simulink library "ddm"  (R2021b)
settings: Solver=VariableStepAuto  StartTime=0.0  StopTime=10.0  RelTol=1e-3
undefined symbols (not defined in the file or in its folder): ENUM_ADASACCSTA_ERROR, ENUM_ADASACCSTA_OFF, ENUM_ADASACCSTA_STANDBY, ENUM_ADASISASTA_OFF, ENUM_ALLOWMOV_ALLOWREADY, ENUM_APS, ENUM_BRKSTA_ERROR, ENUM_BRKSTA_OFF, ENUM_BRKSTA_ON, ENUM_BRKSW_INVALID, ENUM_BRKSW_OFF, ENUM_BRKSW_ON, ENUM_CHGPREACTERRSTA_OBCPRE, ENUM_DCDCFAULTSTA_ANYFAULTLV1, ENUM_DCDCFAULTSTA_ANYFAULTLV2, ENUM_DRIVETRAIN_AWD, ENUM_DRIVETRAIN_FWD, ENUM_DRIVETRAIN_RWD, ENUM_DRSEATSTA_INVALID, ENUM_EDUDRTSTA_NORMAL, ENUM_EPBSTA_APPLIED, ENUM_EPBSTA_RELEASED, ENUM_HVBATTREADYPRE_READY, ENUM_MCUWARN_LV0, ENUM_MCUWARN_LV1, ENUM_MCUWARN_LV2, ENUM_MCUWARN_LV3, ENUM_MCUWARN_NOERROR, ENUM_OBCFAULTSTA_ANYFAULT, ENUM_PAS_R2F2, ENUM_PDFAULT_BATTPDFAIL, ENUM_PDFAULT_DCDCDISABLE, ENUM_PDFAULT_MCUDISABLE, ENUM_PDFAULT_MCUDISCHRG, ENUM_POWERSTA_OFF, ENUM_POWERSTA_ON, ENUM_POWERSTA_READY, ENUM_POWERSTA_STANDBY, ENUM_PRESSINDI_LOW, ENUM_PUFAULT_BATTUPFAIL, ENUM_PUFAULT_DCDCENABLEFAIL, ENUM_PUFAULT_PRECHRGCHKFAIL, ENUM_PUFAULT_SAFETYCHKFAIL, ENUM_PUSTATE_COMPLETED, ENUM_PWRSTASW_OFF, ENUM_PWRSTASW_OFFA, ENUM_PWRSTASW_OFFCHVCHRG, ENUM_PWRSTASW_OFFCLVCHRG, ENUM_PWRSTASW_ON, ENUM_PWRSTASW_ONHVCHRG, ENUM_PWRSTASW_READY, ENUM_PWRSTASW_STANDBY, ENUM_RANGESTA_12IN, ENUM_SHIFTCOMMAND_D, ENUM_SHIFTCOMMAND_N, ENUM_SHIFTCOMMAND_P, ENUM_SHIFTCOMMAND_R, ENUM_VEHMALFUNLV_2ND, ENUM_VEHMALFUNLV_3RD, ENUM_VEHMALFUNLV_4TH ... (+835)
libraries: hcu_lib x750, $bdroot x12, simulink x5
(part 10 of 28)

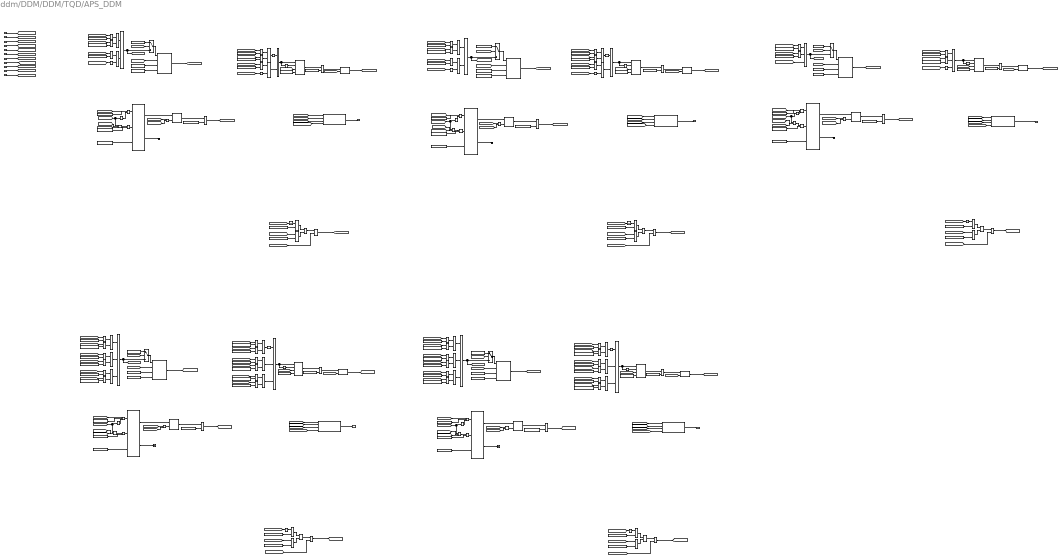
== system ddm/DDM/DDM/TQD/APS_DDM ==
  note: APS2 5V Out of Range (5vAPS2PwrErr)
  note: APS2 Signal Out of Range (APS2SigOoR)
  note: APS Correlation Error (APSCorrErr)
  note: APS1 5V Out of Range (5vAPS1PwrErr)
  note: APS1 Signal Out of Range (APS1SigOoR)
  VPMM_SysPwrSta_enum : Inport
  VINP_AccelPedal1Vol_V : Inport  Port=2
  VINP_AccelPedal2Vol_V : Inport  Port=3
  VDHP_EAPS12RangeSta_enum : Inport  Port=4
  VDHP_EAPCRBAD_flg : Inport  Port=5
  VINP_Pedal1Ref5V_V : Inport  Port=6
  VINP_Pedal2Ref5V_V : Inport  Port=7
  VINP_HVBattSOC_pct : Inport  Port=8
  task_time_s : Inport  Port=9
  DTC_clear_request : Inport  Port=10
  VDDM_AuxBattVolV_V : Inport  Port=11
  Constant{1,10,26,59,94} (5 alike) : Constant  Value=ENUM_POWERSTA_OFF
  Constant{62,65,84,92,100,103} (6 alike) : Constant  Value=ENUM_PWRSTASW_OFF
  Constant101 : Constant  Value=KDDM_APS2SigOoRHiLim_V
  Constant102 : Constant  Value=KDDM_APS2SigOoRLoLim_V
  Constant104 : Constant  Value=KDDM_APS2SigOoRHiLim_V
  Constant105 : Constant  Value=KDDM_APS2SigOoRLoLim_V
  Constant{2,11,76,95,106} (5 alike) : Constant  Value=ENUM_POWERSTA_STANDBY
  Constant107 : Constant  Value=KDDM_APS2SigOoRPassTO_s
  Constant108 : Constant  Value=KDDM_APS2SigOoRPassTO_s
  Constant109 : Constant  Value=KDDM_5vAPS2PwrErrPassTO_s
  Constant110 : Constant  Value=KDDM_APS2SigOoRCFSSW_flg
  Constant{21,85,90,99,111} (5 alike) : Constant  Value=FALSE
  Constant112 : Constant  Value=KDDM_5vAPS2PwrErrDetTO_s
  Constant113 : Constant  Value=KDDM_5vAPS2PwrErrCFSSW_flg
  Constant116 : Constant  Value=KDDM_5vAPS2PwrErrDetSW_flg
  Constant117 : Constant  Value=KDDM_5vAPS2PwrErrPassSW_flg
  Constant118 : Constant  Value=KDDM_5vAPS2PwrErrDTC_cnt
  Constant119 : Constant  Value=KDDM_5vAPS2PwrErrDTC_cnt
  Constant12 : Constant  Value=KDDM_APS1SigOoRDetSW_flg
  Constant13 : Constant  Value=KDDM_APS1SigOoRPassSW_flg
  Constant132 : Constant  Value=KDDM_APS1SigOoRDTC_cnt
  Constant14 : Constant  Value=KDDM_APS1SigOoRDTC_cnt
  Constant15 : Constant  Value=KDDM_APS2SigOoRDTC_cnt
  Constant{16,24,27,35} (4 alike) : Constant  Value=KDDM_LVBattHiLim_V
  Constant{17,28,31,36} (4 alike) : Constant  Value=KDDM_LVBattLoLim_V
  Constant{18,29,32,37} (4 alike) : Constant  Value=ENUM_PWRSTASW_READY
  Constant19 : Constant  Value=KDDM_5vAPS1PwrErrPassTO_s
  Constant20 : Constant  Value=KDDM_5vAPS1PwrErrPassTO_s
  Constant22 : Constant  Value=KDDM_5vAPS1PwrErrDetTO_s
  Constant23 : Constant  Value=KDDM_5vAPS1PwrErrCFSSW_flg
  Constant{7,25,38,41} (4 alike) : Constant  Value=ENUM_PWRSTASW_ON
  Constant3 : Constant  Value=KDDM_5vAPS1PwrErrDetSW_flg
  Constant30 : Constant  Value=KDDM_5vAPS2PwrErrPassTO_s
  Constant{8,33,39,42} (4 alike) : Constant  Value=KDDM_5vAPS1PwrErrHiLim_V
  Constant{9,34,40,43} (4 alike) : Constant  Value=KDDM_5vAPS1PwrErrLoLim_V
  Constant4 : Constant  Value=KDDM_5vAPS1PwrErrPassSW_flg
  Constant5 : Constant  Value=KDDM_5vAPS1PwrErrDTC_cnt
  Constant55 : Constant  Value=KDDM_APSCorrErrPassTO_s
  Constant56 : Constant  Value=ENUM_RANGESTA_12IN
  Constant57 : Constant  Value=KDDM_APSCorrErrDetTO_s
  Constant58 : Constant  Value=KDDM_APSCorrErrDTC_cnt
  Constant6 : Constant  Value=KDDM_5vAPS1PwrErrDTC_cnt
  Constant63 : Constant  Value=KDDM_APS1SigOoRHiLim_V
  Constant64 : Constant  Value=KDDM_APS1SigOoRLoLim_V
  Constant66 : Constant  Value=KDDM_APS1SigOoRHiLim_V
  Constant67 : Constant  Value=KDDM_APS1SigOoRLoLim_V
  Constant68 : Constant  Value=KDDM_APS2SigOoRDetTO_s
  Constant69 : Constant  Value=KDDM_APS1SigOoRPassTO_s
  Constant70 : Constant  Value=KDDM_APS1SigOoRPassTO_s
  Constant71 : Constant  Value=KDDM_APSCorrErrCFSSW_flg
  Constant83 : Constant  Value=ENUM_RANGESTA_12IN
  Constant86 : Constant  Value=KDDM_APS1SigOoRDetTO_s
  Constant87 : Constant  Value=KDDM_APSCorrErrDetSW_flg
  Constant88 : Constant  Value=KDDM_APSCorrErrPassSW_flg
  Constant89 : Constant  Value=KDDM_APSCorrErrDTC_cnt
  Constant91 : Constant  Value=KDDM_APSCorrErrPassTO_s
  Constant93 : Constant  Value=KDDM_APS1SigOoRCFSSW_flg
  Constant96 : Constant  Value=KDDM_APS2SigOoRDetSW_flg
  Constant97 : Constant  Value=KDDM_APS2SigOoRPassSW_flg
  Constant98 : Constant  Value=KDDM_APS2SigOoRDTC_cnt
  DTC_Couter{1..5} (5 alike) : hcu_lib/Basic_Blocks/DTC_Couter
  DTC_Info{,1..4} (5 alike) : hcu_lib/Basic_Blocks/DTC_Info
  Equal{1,3..4,6..7,10..12,14..17,36..37,56..57,66..67,74..75} (20 alike) : RelationalOperator  Operator===  OutDataTypeStr=boolean  RndMeth=Simplest
  Equal{5,13,19,23,26..27,29,31,33,35,60,63} (12 alike) : RelationalOperator  Operator=<  OutDataTypeStr=boolean  RndMeth=Simplest
  Equal{2,8,18,20,22,25,30,32,34,38,59,62} (12 alike) : RelationalOperator  Operator=>  OutDataTypeStr=boolean  RndMeth=Simplest
  Equal{21,24,51,53,58,61} (6 alike) : RelationalOperator  Operator=~=  OutDataTypeStr=boolean  RndMeth=Simplest
  Equal{9,28,55,65,70} (5 alike) : RelationalOperator  OutDataTypeStr=boolean  RndMeth=Simplest
  Logical Operator{1..2,8,10,12..14,19,26..27,33,37,41,48,50,52,54,56,80,97,103,110} (22 alike) : Logic  Operator=OR  AllPortsSameDT=off  OutDataTypeStr=boolean
  Logical Operator{4,6..7,9,16..18,20,24,30..32,34,38..39,47,59,72,82,85,100..102,107..109,116} (27 alike) : Logic  AllPortsSameDT=off  OutDataTypeStr=boolean
  Logical Operator{22,28..29,36,40,42,45,49,51,53,55,62,71,73,83,98,105,111..112} (19 alike) : Logic  Operator=NOT  AllPortsSameDT=off  OutDataTypeStr=boolean
  Logical Operator{11,15,35,43,60} (5 alike) : Logic  Operator=OR  Inputs=3  AllPortsSameDT=off  OutDataTypeStr=boolean
  Logical Operator{3,5,21,23,25,44,46,70,84,86,115} (11 alike) : Logic  Inputs=3  AllPortsSameDT=off  OutDataTypeStr=boolean
  SR_Latch{,1..4,6,12,15,18,20} (10 alike) : hcu_lib/Basic_Blocks/SR_Latch
  Switch{1..4,6} (5 alike) : Switch  Criteria=u2 ~= 0
  Terminator{,1..4} (5 alike) : Terminator
  Test Detection Criteria{1..5} (5 alike) : hcu_lib/Basic_Blocks/Test Detection Criteria
  Timer{1,4..5,13,15} (5 alike) : hcu_lib/Basic_Blocks/Timer
  Unit Delay{,1..2,5,7} (5 alike) : UnitDelay  SampleTime=-1  HasFrameUpgradeWarning=on
  VDDM_APS1SigOoRDTC_raw32 : Outport
  VDDM_APS2SigOoRDTC_raw32 : Outport  Port=2
  VDDM_APSCorrErrDTC_raw32 : Outport  Port=3
  VDDM_5vAPS1PwrErrDTC_raw32 : Outport  Port=4
  VDDM_5vAPS2PwrErrDTC_raw32 : Outport  Port=5
  wires:
  Logical Operator56/1 -> SR_Latch3/2
  [DTC_clear_request] -> Logical Operator56/2
  [DTC_clear_request] -> Logical Operator15/1, Logical Operator55/1
  Logical Operator55/1 -> Logical Operator21/3
  [DTC_clear_request] -> Logical Operator54/2
  Logical Operator54/1 -> SR_Latch1/2
  [DTC_clear_request] -> Logical Operator53/1, Logical Operator11/1
  Logical Operator53/1 -> Logical Operator23/3
  [DTC_clear_request] -> Logical Operator52/2
  Logical Operator52/1 -> SR_Latch12/2
  [DTC_clear_request] -> Logical Operator51/1, Logical Operator60/1
  Logical Operator51/1 -> Logical Operator84/3
  [DTC_clear_request] -> Logical Operator50/2
  Logical Operator50/1 -> SR_Latch6/2
  [DTC_clear_request] -> Logical Operator49/1, Logical Operator43/1
  Logical Operator49/1 -> Logical Operator115/3
  [DTC_clear_request] -> Logical Operator37/2
  Logical Operator37/1 -> SR_Latch/2
  Logical Operator29/1 -> Logical Operator5/3
  [DTC_clear_request] -> Logical Operator29/1, Logical Operator35/1
  Logical Operator45/1 -> Logical Operator46/1
  Logical Operator48/1 -> Logical Operator46/2
  [VPMM_SysPwrSta_enum] -> Equal37/1
  Equal36/1 -> Logical Operator48/1
  Constant43/1 -> Equal35/2
  Constant41/1 -> Equal36/2
  Equal35/1 -> Logical Operator14/2
  Equal34/1 -> Logical Operator14/1
  Equal37/1 -> Logical Operator48/2
  Logical Operator47/1 -> Logical Operator46/3
  Constant29/1 -> Equal37/2
  [VPMM_SysPwrSta_enum] -> Equal36/1
  [VINP_Pedal2Ref5V_V] -> Equal34/1
  Logical Operator14/1 -> Logical Operator45/1
  Equal27/1 -> Logical Operator47/2
  Constant28/1 -> Equal38/2
  Equal38/1 -> Logical Operator47/1
  Constant42/1 -> Equal34/2
  [VINP_Pedal2Ref5V_V] -> Equal35/1
  Constant27/1 -> Equal27/2
  [VDDM_AuxBattVolV_V] -> Equal38/1
  [VDDM_AuxBattVolV_V] -> Equal27/1
  [VDDM_AuxBattVolV_V] -> Equal31/1
  [VDDM_AuxBattVolV_V] -> Equal30/1
  Equal30/1 -> Logical Operator20/1
  Constant35/1 -> Equal31/2
  [VINP_Pedal2Ref5V_V] -> Equal33/1
  Constant36/1 -> Equal30/2
  Constant39/1 -> Equal32/2
  Logical Operator20/1 -> Logical Operator44/3
  Equal17/1 -> Logical Operator26/2
  Equal31/1 -> Logical Operator20/2
  [VINP_Pedal2Ref5V_V] -> Equal32/1
  Constant37/1 -> Equal17/2
  [VPMM_SysPwrSta_enum] -> Equal14/1
  Logical Operator27/1 -> Logical Operator44/1
  Equal32/1 -> Logical Operator27/1
  Equal33/1 -> Logical Operator27/2
  Constant38/1 -> Equal14/2
  Constant40/1 -> Equal33/2
  [VPMM_SysPwrSta_enum] -> Equal17/1
  Equal14/1 -> Logical Operator26/1
  Logical Operator26/1 -> Logical Operator44/2
  Logical Operator22/1 -> Logical Operator25/1
  Logical Operator10/1 -> Logical Operator22/1
  [VDDM_AuxBattVolV_V] -> Equal13/1
  [VDDM_AuxBattVolV_V] -> Equal8/1
  Equal8/1 -> Logical Operator7/1
  Constant16/1 -> Equal13/2
  [VINP_Pedal1Ref5V_V] -> Equal29/1
  Constant17/1 -> Equal8/2
  Constant33/1 -> Equal20/2
  Logical Operator7/1 -> Logical Operator25/3
  Equal7/1 -> Logical Operator8/2
  Equal13/1 -> Logical Operator7/2
  [VINP_Pedal1Ref5V_V] -> Equal20/1
  Constant18/1 -> Equal7/2
  [VPMM_SysPwrSta_enum] -> Equal6/1
  Equal20/1 -> Logical Operator10/1
  Equal29/1 -> Logical Operator10/2
  Constant25/1 -> Equal6/2
  Constant34/1 -> Equal29/2
  [VPMM_SysPwrSta_enum] -> Equal7/1
  Equal6/1 -> Logical Operator8/1
  Logical Operator8/1 -> Logical Operator25/2
  Constant32/1 -> Equal12/2
  [VPMM_SysPwrSta_enum] -> Equal12/1
  Equal12/1 -> Logical Operator19/2
  Logical Operator19/1 -> Logical Operator3/2
  Equal1/1 -> Logical Operator19/1
  Equal18/1 -> Logical Operator18/1
  Equal19/1 -> Logical Operator18/2
  Logical Operator18/1 -> Logical Operator3/3
  Constant31/1 -> Equal18/2
  Constant24/1 -> Equal19/2
  [VDDM_AuxBattVolV_V] -> Equal18/1
  [VDDM_AuxBattVolV_V] -> Equal19/1
  VDDM_AuxBattVolV_V/1 -> [VDDM_AuxBattVolV_V]
  Logical Operator44/1 -> Switch4/3, [VDDM_5vAPS2PwrErrRst_flg]
  DTC_Couter5/1 -> SR_Latch3/1
  Logical Operator16/1 -> Logical Operator13/1
  Logical Operator15/1 -> Logical Operator59/1
  Equal70/1 -> SR_Latch4/1
  Timer5/1 -> Equal70/1
  Test Detection Criteria5/1 -> [VDDM_5vAPS2PwrErrDet_flg]  "VDDM_5vAPS2PwrErrDet_flg"
  Logical Operator62/1 -> Timer5/2
  [VDDM_5vAPS2PwrErrDet_flg] -> Logical Operator21/1
  DTC_Info4/1 -> VDDM_5vAPS2PwrErrDTC_raw32/1  "VDDM_5vAPS2PwrErrDTC_raw32"
  SR_Latch4/1 -> [VDDM_5vAPS2PwrErrPass_flg]  "VDDM_5vAPS2PwrErrPass_flg"
  [VDDM_5vAPS2PwrErrCFSRls_flg] -> Logical Operator15/2
  [VDDM_5vAPS2PwrErrCFS_flg] -> DTC_Info4/3
  Constant116/1 -> Logical Operator21/2
  Logical Operator59/1 -> DTC_Couter5/2
  Constant109/1 -> Timer5/4
  Constant111/1 -> Switch4/1
  [DTC_clear_request] -> DTC_Info4/4
  Constant113/1 -> Logical Operator72/2
  [VPMM_SysPwrSta_enum] -> Equal16/1
  [task_time_s] -> Timer5/3
  Constant26/1 -> Equal15/2
  Constant118/1 -> Test Detection Criteria5/3
  [task_time_s] -> Test Detection Criteria5/2
  Constant119/1 -> DTC_Couter5/3
  Constant106/1 -> Equal16/2
  SR_Latch3/1 -> Logical Operator72/1
  Equal15/1 -> Logical Operator16/1
  [VDDM_5vAPS2PwrErrPass_flg] -> DTC_Info4/2
  Constant30/1 -> Equal70/2
  Unit Delay2/1 -> Equal15/1
  [VPMM_SysPwrSta_enum] -> Unit Delay2/1
  [DTC_clear_request] -> Logical Operator13/2
  [DTC_clear_request] -> Switch4/2
  Logical Operator13/1 -> [VDDM_5vAPS2PwrErrCFSRls_flg]  "VDDM_5vAPS2PwrErrCFSRls_flg"
  Constant117/1 -> Logical Operator59/2
  Constant112/1 -> Test Detection Criteria5/4
  Equal16/1 -> Logical Operator16/2
  [VDDM_5vAPS2PwrErrRst_flg] -> SR_Latch4/2
  [VDDM_5vAPS2PwrErrCFSRls_flg] -> Logical Operator56/1
  Logical Operator21/1 -> DTC_Couter5/1
  Logical Operator72/1 -> [VDDM_5vAPS2PwrErrCFS_flg]  "VDDM_5vAPS2PwrErrCFS_flg"
  DTC_Couter5/2 -> Terminator4/1  "VDDM_5vAPS2PwrErrDTC_cnt"
  Logical Operator46/1 -> Logical Operator62/1, Timer5/1
  [VDDM_5vAPS2PwrErrDet_flg] -> DTC_Info4/1
  Switch4/1 -> Test Detection Criteria5/1
  [VDDM_5vAPS2PwrErrPass_flg] -> Logical Operator15/3
  VINP_HVBattSOC_pct/1 -> [VINP_HVBattSOC_pct]
  [VINP_Pedal1Ref5V_V] -> Equal5/1
  [VINP_Pedal1Ref5V_V] -> Equal2/1
  Logical Operator3/1 -> Switch3/3, [VDDM_5vAPS1PwrErrRst_flg]
  Constant9/1 -> Equal5/2
  [VPMM_SysPwrSta_enum] -> Equal1/1
  Constant8/1 -> Equal2/2
  Logical Operator2/1 -> Logical Operator3/1
  Equal5/1 -> Logical Operator2/2
  Equal2/1 -> Logical Operator2/1
  Constant7/1 -> Equal1/2
  Logical Operator1/1 -> [VDDM_5vAPS1PwrErrCFSRls_flg]  "VDDM_5vAPS1PwrErrCFSRls_flg"
  Logical Operator17/1 -> Logical Operator1/1
  SR_Latch2/1 -> [VDDM_5vAPS1PwrErrPass_flg]  "VDDM_5vAPS1PwrErrPass_flg"
  Logical Operator9/1 -> [VDDM_5vAPS1PwrErrCFS_flg]  "VDDM_5vAPS1PwrErrCFS_flg"
  Constant21/1 -> Switch3/1
  Logical Operator25/1 -> Logical Operator40/1, Timer4/1
  [task_time_s] -> Timer4/3
  Switch3/1 -> Test Detection Criteria2/1
  DTC_Info3/1 -> VDDM_5vAPS1PwrErrDTC_raw32/1  "VDDM_5vAPS1PwrErrDTC_raw32"
  [VPMM_SysPwrSta_enum] -> Equal11/1
  [DTC_clear_request] -> DTC_Info3/4
  Constant6/1 -> DTC_Couter4/3
  [task_time_s] -> Test Detection Criteria2/2
  [VPMM_SysPwrSta_enum] -> Unit Delay1/1
  SR_Latch1/1 -> Logical Operator9/1
  Equal10/1 -> Logical Operator17/1
  Constant2/1 -> Equal11/2
  Constant1/1 -> Equal10/2
  Constant5/1 -> Test Detection Criteria2/3
  DTC_Couter4/2 -> Terminator3/1  "VDDM_5vAPS1PwrErrDTC_cnt"
  [VDDM_5vAPS1PwrErrPass_flg] -> DTC_Info3/2
  [DTC_clear_request] -> Logical Operator1/2
  Logical Operator23/1 -> DTC_Couter4/1
  Constant19/1 -> Equal9/2
  Unit Delay1/1 -> Equal10/1
  Constant4/1 -> Logical Operator24/2
  Constant3/1 -> Logical Operator23/2
  [DTC_clear_request] -> Switch3/2
  [VDDM_5vAPS1PwrErrPass_flg] -> Logical Operator11/3
  DTC_Couter4/1 -> SR_Latch1/1
  Test Detection Criteria2/1 -> [VDDM_5vAPS1PwrErrDet_flg]  "VDDM_5vAPS1PwrErrDet_flg"
  Logical Operator11/1 -> Logical Operator24/1
  Equal11/1 -> Logical Operator17/2
  Logical Operator24/1 -> DTC_Couter4/2
  [VDDM_5vAPS1PwrErrCFSRls_flg] -> Logical Operator11/2
  Equal9/1 -> SR_Latch2/1
  Logical Operator40/1 -> Timer4/2
  Constant20/1 -> Timer4/4
  Timer4/1 -> Equal9/1
  [VDDM_5vAPS1PwrErrDet_flg] -> Logical Operator23/1
  Constant23/1 -> Logical Operator9/2
  Constant22/1 -> Test Detection Criteria2/4
  [VDDM_5vAPS1PwrErrRst_flg] -> SR_Latch2/2
  [VDDM_5vAPS1PwrErrDet_flg] -> DTC_Info3/1
  [VDDM_5vAPS1PwrErrCFS_flg] -> DTC_Info3/3
  [VDDM_5vAPS1PwrErrCFSRls_flg] -> Logical Operator54/1
  VINP_Pedal2Ref5V_V/1 -> [VINP_Pedal2Ref5V_V]
  VINP_Pedal1Ref5V_V/1 -> [VINP_Pedal1Ref5V_V]
  [VDDM_APSCorrErrRst_flg] -> SR_Latch20/2
  [VDDM_APS2SigOoRRst_flg] -> SR_Latch15/2
  [VDDM_APS1SigOoRRst_flg] -> SR_Latch18/2
  Logical Operator60/1 -> Logical Operator85/1
  [VDDM_APSCorrErrPass_flg] -> Logical Operator60/3
  [VDDM_APSCorrErrCFSRls_flg] -> Logical Operator60/2
  Logical Operator43/1 -> Logical Operator116/1
  [VDDM_APS2SigOoRPass_flg] -> Logical Operator43/3
  [VDDM_APS2SigOoRCFSRls_flg] -> Logical Operator43/2
  Logical Operator35/1 -> Logical Operator6/1
  [VDDM_APS1SigOoRCFSRls_flg] -> Logical Operator35/2
  [VDDM_APS1SigOoRPass_flg] -> Logical Operator35/3
  Constant99/1 -> Switch2/1
  Logical Operator86/1 -> Switch2/3, [VDDM_APSCorrErrRst_flg]
  Switch2/1 -> Test Detection Criteria1/1
  [DTC_clear_request] -> Switch2/2
  Constant90/1 -> Switch1/1
  Logical Operator101/1 -> Switch1/3, [VDDM_APS2SigOoRRst_flg]
  Switch1/1 -> Test Detection Criteria4/1
  [DTC_clear_request] -> Switch1/2
  Constant85/1 -> Switch6/1
  Logical Operator31/1 -> Switch6/3, [VDDM_APS1SigOoRRst_flg]
  Switch6/1 -> Test Detection Criteria3/1
  [DTC_clear_request] -> Switch6/2
  [DTC_clear_request] -> DTC_Info2/4
  [DTC_clear_request] -> DTC_Info1/4
  [DTC_clear_request] -> DTC_Info/4
  Logical Operator34/1 -> [VDDM_APSCorrErrCFS_flg]  "VDDM_APSCorrErrCFS_flg"
  SR_Latch12/1 -> Logical Operator34/1
  Constant71/1 -> Logical Operator34/2
  VDHP_EAPCRBAD_flg/1 -> [VDHP_EAPCRBAD_flg]
  VDHP_EAPS12RangeSta_enum/1 -> [VDHP_EAPS12RangeSta_enum]
  DTC_Info2/1 -> VDDM_APSCorrErrDTC_raw32/1  "VDDM_APSCorrErrDTC_raw32"
  [VDDM_APSCorrErrCFS_flg] -> DTC_Info2/3
  DTC_Couter3/2 -> Terminator2/1  "VDDM_APSCorrErrDTC_cnt"
  DTC_Couter3/1 -> SR_Latch12/1
  Constant89/1 -> DTC_Couter3/3
  Constant58/1 -> Test Detection Criteria1/3
  VINP_AccelPedal2Vol_V/1 -> [VINP_AccelPedal2Vol_V]
  VINP_AccelPedal1Vol_V/1 -> [VINP_AccelPedal1Vol_V]
  VPMM_SysPwrSta_enum/1 -> [VPMM_SysPwrSta_enum]
  DTC_Info1/1 -> VDDM_APS2SigOoRDTC_raw32/1  "VDDM_APS2SigOoRDTC_raw32"
  [VDDM_APS2SigOoRCFS_flg] -> DTC_Info1/3
  SR_Latch6/1 -> Logical Operator102/1
  [VDDM_APS2SigOoRCFSRls_flg] -> Logical Operator50/1
  DTC_Couter2/1 -> SR_Latch6/1
  DTC_Couter2/2 -> Terminator1/1  "VDDM_APS2SigOoRDTC_cnt"
  Constant98/1 -> DTC_Couter2/3
  Logical Operator116/1 -> DTC_Couter2/2
  Logical Operator115/1 -> DTC_Couter2/1
  Constant68/1 -> Test Detection Criteria4/4
  Constant15/1 -> Test Detection Criteria4/3
  [task_time_s] -> Test Detection Criteria4/2
  DTC_Couter1/2 -> Terminator/1  "VDDM_APS1SigOoRDTC_cnt"
  Equal28/1 -> SR_Latch18/1
  Logical Operator39/1 -> Logical Operator73/1, Timer1/1
  [VDDM_APS1SigOoRCFSRls_flg] -> Logical Operator37/1
  DTC_Couter1/1 -> SR_Latch/1
  Constant14/1 -> DTC_Couter1/3
  Logical Operator6/1 -> DTC_Couter1/2
  Logical Operator5/1 -> DTC_Couter1/1
  DTC_Info/1 -> VDDM_APS1SigOoRDTC_raw32/1  "VDDM_APS1SigOoRDTC_raw32"
  [VDDM_APS1SigOoRPass_flg] -> DTC_Info/2
  [VDDM_APS1SigOoRCFS_flg] -> DTC_Info/3
  Test Detection Criteria3/1 -> [VDDM_APS1SigOoRDet_flg]  "VDDM_APS1SigOoRDet_flg"
  Constant132/1 -> Test Detection Criteria3/3
  Constant86/1 -> Test Detection Criteria3/4
  [task_time_s] -> Test Detection Criteria3/2
  Logical Operator71/1 -> Logical Operator70/3
  [VDHP_EAPCRBAD_flg] -> Logical Operator71/1
  Constant84/1 -> Equal53/2
  [VPMM_SysPwrSta_enum] -> Equal53/1
  Constant56/1 -> Equal75/2
  Logical Operator70/1 -> Timer13/1, Logical Operator83/1
  [VDHP_EAPS12RangeSta_enum] -> Equal75/1
  Equal53/1 -> Logical Operator70/1
  Equal75/1 -> Logical Operator70/2
  Constant83/1 -> Equal74/2
  Equal74/1 -> Logical Operator86/2
  [VDHP_EAPS12RangeSta_enum] -> Equal74/1
  Equal55/1 -> SR_Latch20/1
  SR_Latch20/1 -> [VDDM_APSCorrErrPass_flg]  "VDDM_APSCorrErrPass_flg"
  [VDDM_5vAPS2PwrErrCFS_flg] -> Logical Operator98/1
  Logical Operator97/1 -> [VDDM_APS2SigOoRCFSRls_flg]  "VDDM_APS2SigOoRCFSRls_flg"
  [VINP_AccelPedal2Vol_V] -> Equal60/1
  [task_time_s] -> Timer15/3
  SR_Latch15/1 -> [VDDM_APS2SigOoRPass_flg]  "VDDM_APS2SigOoRPass_flg"
  Equal66/1 -> Logical Operator109/1
  Unit Delay7/1 -> Equal66/1
  Equal65/1 -> SR_Latch15/1
  [VDDM_APS2SigOoRDet_flg] -> Logical Operator115/1
  [VDDM_5vAPS2PwrErrCFS_flg] -> Logical Operator105/1
  Logical Operator105/1 -> Logical Operator107/2
  Constant105/1 -> Equal63/2
  [VINP_AccelPedal2Vol_V] -> Equal59/1
  [VINP_AccelPedal2Vol_V] -> Equal62/1
  Constant102/1 -> Equal60/2
  [VPMM_SysPwrSta_enum] -> Equal58/1
  [VPMM_SysPwrSta_enum] -> Equal61/1
  Equal60/1 -> Logical Operator103/2
  [VINP_AccelPedal2Vol_V] -> Equal63/1
  Equal63/1 -> Logical Operator110/2
  Timer15/1 -> Equal65/1
  Logical Operator112/1 -> Timer15/2
  Constant103/1 -> Equal61/2
  Constant108/1 -> Timer15/4
  Logical Operator111/1 -> Logical Operator108/1
  Equal62/1 -> Logical Operator110/1
  [VPMM_SysPwrSta_enum] -> Equal67/1
  Logical Operator102/1 -> [VDDM_APS2SigOoRCFS_flg]  "VDDM_APS2SigOoRCFS_flg"
  Constant110/1 -> Logical Operator102/2
  [VPMM_SysPwrSta_enum] -> Unit Delay7/1
  Constant107/1 -> Equal65/2
  Constant97/1 -> Logical Operator116/2
  Constant100/1 -> Equal58/2
  Constant96/1 -> Logical Operator115/2
  Equal59/1 -> Logical Operator103/1
  Logical Operator98/1 -> Logical Operator100/2
  Logical Operator110/1 -> Logical Operator111/1
  Constant104/1 -> Equal62/2
  Logical Operator109/1 -> Logical Operator97/1
  Constant101/1 -> Equal59/2
  Test Detection Criteria4/1 -> [VDDM_APS2SigOoRDet_flg]  "VDDM_APS2SigOoRDet_flg"
  Constant94/1 -> Equal66/2
  Equal58/1 -> Logical Operator100/1
  Logical Operator103/1 -> Logical Operator101/1
  Equal61/1 -> Logical Operator107/1
  Logical Operator107/1 -> Logical Operator108/2
  Equal67/1 -> Logical Operator109/2
  Logical Operator100/1 -> Logical Operator101/2
  Logical Operator108/1 -> Timer15/1, Logical Operator112/1
  Constant95/1 -> Equal67/2
  [DTC_clear_request] -> Logical Operator97/2
  SR_Latch18/1 -> [VDDM_APS1SigOoRPass_flg]  "VDDM_APS1SigOoRPass_flg"
  Constant93/1 -> Logical Operator32/2
  Logical Operator32/1 -> [VDDM_APS1SigOoRCFS_flg]  "VDDM_APS1SigOoRCFS_flg"
  SR_Latch/1 -> Logical Operator32/1
  [VDHP_EAPCRBAD_flg] -> Logical Operator86/3
  [VPMM_SysPwrSta_enum] -> Equal51/1
  Constant92/1 -> Equal51/2
  Equal51/1 -> Logical Operator86/1
  Constant76/1 -> Equal57/2
  Constant55/1 -> Timer13/4
  Constant87/1 -> Logical Operator84/2
  Logical Operator80/1 -> [VDDM_APSCorrErrCFSRls_flg]  "VDDM_APSCorrErrCFSRls_flg"
  [VDDM_APSCorrErrCFSRls_flg] -> Logical Operator52/1
  Logical Operator82/1 -> Logical Operator80/1
  [task_time_s] -> Test Detection Criteria1/2
  Constant91/1 -> Equal55/2
  Unit Delay5/1 -> Equal56/1
  Test Detection Criteria1/1 -> [VDDM_APSCorrErrDet_flg]  "VDDM_APSCorrErrDet_flg"
  Logical Operator83/1 -> Timer13/2
  Logical Operator84/1 -> DTC_Couter3/1
  Logical Operator85/1 -> DTC_Couter3/2
  Timer13/1 -> Equal55/1
  Constant88/1 -> Logical Operator85/2
  [VDDM_APSCorrErrDet_flg] -> Logical Operator84/1
  Constant59/1 -> Equal56/2
  [task_time_s] -> Timer13/3
  Constant57/1 -> Test Detection Criteria1/4
  [DTC_clear_request] -> Logical Operator80/2
  Equal57/1 -> Logical Operator82/2
  Equal56/1 -> Logical Operator82/1
  [VPMM_SysPwrSta_enum] -> Unit Delay5/1
  [VPMM_SysPwrSta_enum] -> Equal57/1
  [task_time_s] -> Timer1/3
  Constant70/1 -> Timer1/4
  Timer1/1 -> Equal28/1
  Constant69/1 -> Equal28/2
  Logical Operator73/1 -> Timer1/2
  Logical Operator42/1 -> Logical Operator39/1
  Logical Operator38/1 -> Logical Operator39/2
  Logical Operator36/1 -> Logical Operator38/2
  Equal24/1 -> Logical Operator38/1
  [VDDM_5vAPS1PwrErrCFS_flg] -> Logical Operator36/1
  Constant65/1 -> Equal24/2
  [VPMM_SysPwrSta_enum] -> Equal24/1
  Equal26/1 -> Logical Operator41/2
  Equal25/1 -> Logical Operator41/1
  Constant67/1 -> Equal26/2
  Constant66/1 -> Equal25/2
  [VINP_AccelPedal1Vol_V] -> Equal26/1
  [VINP_AccelPedal1Vol_V] -> Equal25/1
  Logical Operator41/1 -> Logical Operator42/1
  Logical Operator33/1 -> Logical Operator31/1
  [VINP_AccelPedal1Vol_V] -> Equal22/1
  [VINP_AccelPedal1Vol_V] -> Equal23/1
  Constant63/1 -> Equal22/2
  Constant64/1 -> Equal23/2
  Equal22/1 -> Logical Operator33/1
  Equal23/1 -> Logical Operator33/2
  [VPMM_SysPwrSta_enum] -> Equal21/1
  Constant62/1 -> Equal21/2
  [VDDM_5vAPS1PwrErrCFS_flg] -> Logical Operator28/1
  Equal21/1 -> Logical Operator30/1
  Logical Operator28/1 -> Logical Operator30/2
  Logical Operator30/1 -> Logical Operator31/2
  Logical Operator12/1 -> [VDDM_APS1SigOoRCFSRls_flg]  "VDDM_APS1SigOoRCFSRls_flg"
  Logical Operator4/1 -> Logical Operator12/1
  [DTC_clear_request] -> Logical Operator12/2
  Constant13/1 -> Logical Operator6/2
  Constant12/1 -> Logical Operator5/2
  [VDDM_APS1SigOoRDet_flg] -> Logical Operator5/1
  Equal4/1 -> Logical Operator4/2
  Equal3/1 -> Logical Operator4/1
  [VPMM_SysPwrSta_enum] -> Equal4/1
  Constant11/1 -> Equal4/2
  Constant10/1 -> Equal3/2
  Unit Delay/1 -> Equal3/1
  [VPMM_SysPwrSta_enum] -> Unit Delay/1
  task_time_s/1 -> [task_time_s]
  DTC_clear_request/1 -> [DTC_clear_request]
  [VDDM_APS1SigOoRDet_flg] -> DTC_Info/1
  [VDDM_APS2SigOoRDet_flg] -> DTC_Info1/1
  [VDDM_APS2SigOoRPass_flg] -> DTC_Info1/2
  [VDDM_APSCorrErrDet_flg] -> DTC_Info2/1
  [VDDM_APSCorrErrPass_flg] -> DTC_Info2/2

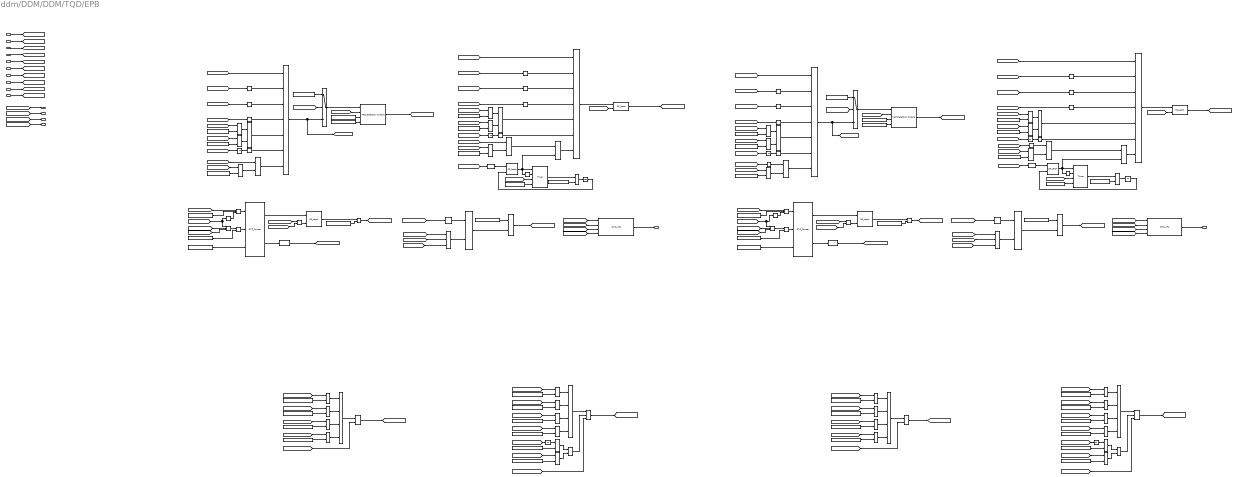
== system ddm/DDM/DDM/TQD/EPB ==
  note: EPB Release Response Timeout (EPBUnlockTO)
  note: EPB Apply Response Timeout (EPBLockTO)
  NO_CAN1_BUS_OFF : Inport
  CAN_LossOfEPB1 : Inport  Port=2
  RC_LossErrOfEPB1 : Inport  Port=3
  CS_LossErrOfEPB1 : Inport  Port=4
  VPMM_SysPwrSta_enum : Inport  Port=5
  VTQD_ActParkRequest_flg : Inport  Port=6
  VINP_EPBSta_enum : Inport  Port=7
  VINP_ShifterHandleCmd_enum : Inport  Port=8
  task_time_s : Inport  Port=9
  DTC_clear_request : Inport  Port=10
  AND{,1..5} (6 alike) : Logic  AllPortsSameDT=off  OutDataTypeStr=boolean
  Constant{,3,23,25} (4 alike) : Constant  Value=ENUM_PWRSTASW_ON
  Constant1 : Constant  Value=KDDM_EPBLockTOCFSSW_flg
  Constant{8,10,26,49} (4 alike) : Constant  Value=ENUM_PWRSTASW_READY
  Constant11 : Constant  Value=ENUM_EPBSTA_RELEASED
  Constant12 : Constant  Value=ENUM_POWERSTA_OFF
  Constant13 : Constant  Value=ENUM_POWERSTA_STANDBY
  Constant{14,29,41,45} (4 alike) : Constant  Value=ENUM_SHIFTCOMMAND_P
  Constant15 : Constant  Value=KDDM_EPBLockTODTC_cnt
  Constant16 : Constant  Value=KDDM_EPBLockTODFSSW_flg
  Constant{17,32,42,46} (4 alike) : Constant  Value=ENUM_SHIFTCOMMAND_N
  Constant{4,18,33,40} (4 alike) : Constant  Value=ENUM_SHIFTCOMMAND_D
  Constant{5,19,34,43} (4 alike) : Constant  Value=ENUM_SHIFTCOMMAND_R
  Constant2 : Constant  Value=FALSE
  Constant20 : Constant  Value=KDDM_EPBLockTODTC_cnt
  Constant21 : Constant  Value=KDDM_EPBUnlockTOPassTO_s
  Constant22 : Constant  Value=KDDM_EPBLockTODetTO_s
  Constant24 : Constant  Value=KDDM_EPBUnlockTOCFSSW_flg
  Constant27 : Constant  Value=ENUM_POWERSTA_OFF
  Constant28 : Constant  Value=ENUM_POWERSTA_STANDBY
  Constant30 : Constant  Value=KDDM_EPBUnlockTODTC_cnt
  Constant31 : Constant  Value=KDDM_EPBUnlockTODFSSW_flg
  Constant35 : Constant  Value=FALSE
  Constant36 : Constant  Value=KDDM_EPBUnlockTODTC_cnt
  Constant38 : Constant  Value=KDDM_EPBUnlockTODetTO_s
  Constant39 : Constant  Value=ENUM_EPBSTA_RELEASED
  Constant44 : Constant  Value=KDDM_EPBUnlockTODetSW_flg
  Constant47 : Constant  Value=KDDM_EPBUnlockTOPassSW_flg
  Constant50 : Constant  Value=ENUM_EPBSTA_APPLIED
  Constant51 : Constant  Value=ENUM_EPBSTA_APPLIED
  Constant52 : Constant  Value=KDDM_EPBLockTOPassTO_s
  Constant53 : Constant  Value=KDDM_EPBUnlockTOPassTO_s
  Constant6 : Constant  Value=KDDM_EPBLockTODetSW_flg
  Constant7 : Constant  Value=KDDM_EPBLockTOPassSW_flg
  Constant9 : Constant  Value=KDDM_EPBLockTOPassTO_s
  DTC_Couter1 : hcu_lib/Basic_Blocks/DTC_Couter
  DTC_Couter2 : hcu_lib/Basic_Blocks/DTC_Couter
  DTC_Info : hcu_lib/Basic_Blocks/DTC_Info
  DTC_Info1 : hcu_lib/Basic_Blocks/DTC_Info
  Data Type Conversion1 : DataTypeConversion  OutDataTypeStr=uint8
  Data Type Conversion2 : DataTypeConversion  OutDataTypeStr=uint8
  Detect Decrease : simulink/Logic and Bit Operations/Detect Decrease  vinit=0.0  OutDataTypeStr=boolean
  Detect Increase1 : simulink/Logic and Bit Operations/Detect Increase  vinit=0.0  OutDataTypeStr=boolean
  Equal{,1..2,4,6,8..26,28,30..34} (30 alike) : RelationalOperator  Operator===  OutDataTypeStr=boolean  RndMeth=Simplest
  Equal27 : RelationalOperator  Operator=~=  OutDataTypeStr=boolean  RndMeth=Simplest
  Equal3 : RelationalOperator  OutDataTypeStr=boolean  RndMeth=Simplest
  Equal5 : RelationalOperator  Operator=~=  OutDataTypeStr=boolean  RndMeth=Simplest
  Equal7 : RelationalOperator  OutDataTypeStr=boolean  RndMeth=Simplest
  Logical Operator{,4,6,8,25,29,49,51} (8 alike) : Logic  Operator=OR  AllPortsSameDT=off  OutDataTypeStr=boolean
  Logical Operator{1..2,9,16..18,24,55} (8 alike) : Logic  AllPortsSameDT=off  OutDataTypeStr=boolean
  Logical Operator{10..11,20,27,37,77} (6 alike) : Logic  Operator=OR  Inputs=3  AllPortsSameDT=off  OutDataTypeStr=boolean
  Logical Operator{12,14,23,28,30..36,38..39,41..48,50} (22 alike) : Logic  Operator=NOT  AllPortsSameDT=off  OutDataTypeStr=boolean
  Logical Operator13 : Logic  Inputs=3  AllPortsSameDT=off  OutDataTypeStr=boolean
  Logical Operator15 : Logic  Inputs=3  AllPortsSameDT=off  OutDataTypeStr=boolean
  Logical Operator{3,5,19,21} (4 alike) : Logic  Inputs=7  AllPortsSameDT=off  OutDataTypeStr=boolean
  Logical Operator{7,22,26,40} (4 alike) : Logic  Operator=OR  Inputs=4  AllPortsSameDT=off  OutDataTypeStr=boolean
  Relay1 : Relay  OnSwitchValue=ONE_INT  OffSwitchValue=ZERO_INT
  Relay2 : Relay  OnSwitchValue=ONE_INT  OffSwitchValue=ZERO_INT
  SR_Latch{1..8} (8 alike) : hcu_lib/Basic_Blocks/SR_Latch
  Switch1 : Switch  Criteria=u2 ~= 0
  Switch6 : Switch  Criteria=u2 ~= 0
  Test Detection Criteria1 : hcu_lib/Basic_Blocks/Test Detection Criteria
  Test Detection Criteria2 : hcu_lib/Basic_Blocks/Test Detection Criteria
  Timer2 : hcu_lib/Basic_Blocks/Timer
  Timer3 : hcu_lib/Basic_Blocks/Timer
  Unit Delay{,1..7} (8 alike) : UnitDelay  SampleTime=-1  HasFrameUpgradeWarning=on
  VDDM_EPBLockTODTC_raw32 : Outport
  VDDM_EPBUnlockTODTC_raw32 : Outport  Port=2
  VDDM_EPBLockTODFS_flg : Outport  Port=3
  VDDM_EPBLockTOCFS_flg : Outport  Port=4
  VDDM_EPBUnlockTODFS_flg : Outport  Port=5
  VDDM_EPBUnlockTOCFS_flg : Outport  Port=6
  wires:
  [DTC_clear_request] -> Logical Operator27/3
  [DTC_clear_request] -> Logical Operator51/2
  Logical Operator51/1 -> SR_Latch3/2
  [DTC_clear_request] -> Logical Operator50/1, Logical Operator10/1
  Logical Operator50/1 -> Logical Operator13/3
  [DTC_clear_request] -> Logical Operator77/3
  [DTC_clear_request] -> Logical Operator49/2
  Logical Operator49/1 -> SR_Latch1/2
  [DTC_clear_request] -> Logical Operator48/1, Logical Operator11/1
  Logical Operator48/1 -> Logical Operator15/3
  Unit Delay7/1 -> SR_Latch8/2
  Unit Delay6/1 -> SR_Latch7/2
  Logical Operator46/1 -> Logical Operator21/3
  [CS_LossErrOfEPB1] -> Logical Operator47/1
  Logical Operator47/1 -> Logical Operator21/4
  Logical Operator45/1 -> Logical Operator21/2
  [RC_LossErrOfEPB1] -> Logical Operator46/1
  [CAN_LossOfEPB1] -> Logical Operator45/1
  Logical Operator43/1 -> Logical Operator19/3
  [CS_LossErrOfEPB1] -> Logical Operator44/1
  Logical Operator44/1 -> Logical Operator19/4
  Logical Operator42/1 -> Logical Operator19/2
  [RC_LossErrOfEPB1] -> Logical Operator43/1
  [CAN_LossOfEPB1] -> Logical Operator42/1
  [CS_LossErrOfEPB1] -> Logical Operator41/1
  [RC_LossErrOfEPB1] -> Logical Operator39/1
  [CAN_LossOfEPB1] -> Logical Operator38/1
  Logical Operator41/1 -> Logical Operator5/4
  Logical Operator38/1 -> Logical Operator5/2
  Logical Operator39/1 -> Logical Operator5/3
  [RC_LossErrOfEPB1] -> Logical Operator35/1
  [CAN_LossOfEPB1] -> Logical Operator12/1
  Logical Operator35/1 -> Logical Operator3/3
  Logical Operator12/1 -> Logical Operator3/2
  Logical Operator36/1 -> Logical Operator3/4
  [CS_LossErrOfEPB1] -> Logical Operator36/1
  AND3/1 -> AND5/1
  AND5/1 -> Logical Operator21/7
  Logical Operator21/1 -> SR_Latch4/1
  Detect Decrease/1 -> SR_Latch8/1
  Constant53/1 -> Equal7/2
  SR_Latch8/1 -> Timer2/1, Logical Operator14/1, AND5/2
  [VTQD_ActParkRequest_flg] -> Detect Decrease/1
  Timer2/1 -> Equal7/1
  Equal7/1 -> Unit Delay7/1
  Constant21/1 -> Timer2/4
  [task_time_s] -> Timer2/3
  Logical Operator14/1 -> Timer2/2
  [VDDM_EPBLockTORst_flg] -> SR_Latch6/2
  SR_Latch6/1 -> [VDDM_EPBLockTOPass_flg]  "VDDM_EPBLockTOPass_flg"
  Logical Operator5/1 -> SR_Latch6/1
  AND1/1 -> Logical Operator5/7
  AND4/1 -> AND1/1
  Equal3/1 -> Unit Delay6/1
  Logical Operator34/1 -> Timer3/2
  SR_Latch7/1 -> Timer3/1, Logical Operator34/1, AND1/2
  Constant9/1 -> Equal3/2
  Timer3/1 -> Equal3/1
  Constant52/1 -> Timer3/4
  [task_time_s] -> Timer3/3
  [VTQD_ActParkRequest_flg] -> Detect Increase1/1
  Detect Increase1/1 -> SR_Latch7/1
  Constant51/1 -> Equal32/2
  Equal32/1 -> AND4/2
  [VTQD_ActParkRequest_flg] -> AND4/1
  [VINP_EPBSta_enum] -> Equal32/1
  DTC_clear_request/1 -> [DTC_clear_request]
  task_time_s/1 -> [task_time_s]
  VINP_ShifterHandleCmd_enum/1 -> [VINP_ShifterHandleCmd_enum]
  VINP_EPBSta_enum/1 -> [VINP_EPBSta_enum]
  VTQD_ActParkRequest_flg/1 -> [VTQD_ActParkRequest_flg]
  VPMM_SysPwrSta_enum/1 -> [VPMM_SysPwrSta_enum]
  CS_LossErrOfEPB1/1 -> [CS_LossErrOfEPB1]
  RC_LossErrOfEPB1/1 -> [RC_LossErrOfEPB1]
  CAN_LossOfEPB1/1 -> [CAN_LossOfEPB1]
  NO_CAN1_BUS_OFF/1 -> [NO_CAN1_BUS_OFF]
  [VTQD_ActParkRequest_flg] -> Logical Operator33/1
  Constant39/1 -> Equal23/2
  Equal23/1 -> AND3/2
  [VINP_EPBSta_enum] -> Equal23/1
  Logical Operator33/1 -> AND3/1
  Logical Operator32/1 -> AND2/1
  [VTQD_ActParkRequest_flg] -> Logical Operator32/1
  AND2/1 -> Logical Operator19/7
  [VINP_EPBSta_enum] -> Equal5/1
  Equal5/1 -> AND2/2
  Constant11/1 -> Equal5/2
  [VTQD_ActParkRequest_flg] -> AND/1
  Equal27/1 -> AND/2
  Constant50/1 -> Equal27/2
  [VINP_EPBSta_enum] -> Equal27/1
  Logical Operator19/1 -> Switch1/3, [VDDM_EPBUnlockTORst_flg]
  [VDDM_EPBLockTOCFS_flg] -> Unit Delay5/1
  Unit Delay5/1 -> Logical Operator23/1
  Logical Operator23/1 -> Logical Operator21/6
  [VPMM_SysPwrSta_enum] -> Equal26/1
  [VPMM_SysPwrSta_enum] -> Equal22/1
  Equal26/1 -> Logical Operator29/2
  [NO_CAN1_BUS_OFF] -> Logical Operator21/1
  Logical Operator29/1 -> Logical Operator21/5
  Equal22/1 -> Logical Operator29/1
  Constant26/1 -> Equal26/2
  Constant25/1 -> Equal22/2
  Constant23/1 -> Equal15/2
  Equal15/1 -> Logical Operator8/1
  Constant49/1 -> Equal16/2
  Equal16/1 -> Logical Operator8/2
  Logical Operator8/1 -> Logical Operator19/5
  [VPMM_SysPwrSta_enum] -> Equal15/1
  [NO_CAN1_BUS_OFF] -> Logical Operator19/1
  [VPMM_SysPwrSta_enum] -> Equal16/1
  [VDDM_EPBLockTOCFS_flg] -> Unit Delay3/1
  Unit Delay3/1 -> Logical Operator28/1
  Logical Operator28/1 -> Logical Operator19/6
  Constant3/1 -> Equal2/2
  Equal2/1 -> Logical Operator4/1
  Constant10/1 -> Equal4/2
  Equal4/1 -> Logical Operator4/2
  Logical Operator4/1 -> Logical Operator5/5
  [VPMM_SysPwrSta_enum] -> Equal2/1
  [NO_CAN1_BUS_OFF] -> Logical Operator5/1
  [VPMM_SysPwrSta_enum] -> Equal4/1
  [VDDM_EPBUnlockTOCFS_flg] -> Unit Delay2/1
  Unit Delay2/1 -> Logical Operator31/1
  Logical Operator31/1 -> Logical Operator5/6
  AND/1 -> Logical Operator3/7
  Unit Delay/1 -> Logical Operator30/1
  Logical Operator30/1 -> Logical Operator3/6
  [VDDM_EPBUnlockTOPass_flg] -> DTC_Info1/2
  Constant29/1 -> Equal18/2
  [VDDM_EPBUnlockTORst_flg] -> SR_Latch4/2
  [VINP_ShifterHandleCmd_enum] -> Equal21/1
  Constant24/1 -> Logical Operator18/2
  [task_time_s] -> Test Detection Criteria2/2
  [VINP_ShifterHandleCmd_enum] -> Equal19/1
  Equal18/1 -> Logical Operator26/1
  Logical Operator26/1 -> Logical Operator25/1
  Constant35/1 -> Switch1/1
  Constant47/1 -> Logical Operator17/2
  [VINP_ShifterHandleCmd_enum] -> Equal18/1
  Constant43/1 -> Equal30/2
  Logical Operator25/1 -> [VDDM_EPBUnlockTODFSRls_flg]  "VDDM_EPBUnlockTODFSRls_flg"
  [VPMM_SysPwrSta_enum] -> Unit Delay1/1
  Equal19/1 -> Logical Operator26/2
  Constant34/1 -> Equal21/2
  [VDDM_EPBUnlockTOPass_flg] -> Logical Operator25/2
  Test Detection Criteria2/1 -> [VDDM_EPBUnlockTODet_flg]  "VDDM_EPBUnlockTODet_flg"
  [VPMM_SysPwrSta_enum] -> Equal17/1
  Constant32/1 -> Equal19/2
  [VINP_ShifterHandleCmd_enum] -> Equal20/1
  [VINP_ShifterHandleCmd_enum] -> Equal28/1
  Constant28/1 -> Equal17/2
  Logical Operator27/1 -> SR_Latch5/2
  Logical Operator9/1 -> Logical Operator20/2
  Equal20/1 -> Logical Operator26/3
  Constant42/1 -> Equal25/2
  [VINP_ShifterHandleCmd_enum] -> Equal30/1
  Logical Operator20/1 -> [VDDM_EPBUnlockTOCFSRls_flg]  "VDDM_EPBUnlockTOCFSRls_flg"
  [VDDM_EPBUnlockTODet_flg] -> Logical Operator13/1
  Equal21/1 -> Logical Operator26/4
  Constant40/1 -> Equal28/2
  Equal28/1 -> Logical Operator22/3
  Constant33/1 -> Equal20/2
  [VINP_ShifterHandleCmd_enum] -> Equal24/1
  Equal31/1 -> Logical Operator9/1
  Logical Operator22/1 -> Logical Operator20/1
  SR_Latch3/1 -> Logical Operator18/1
  Equal25/1 -> Logical Operator22/2
  Constant27/1 -> Equal31/2
  Equal17/1 -> Logical Operator9/2
  Constant30/1 -> DTC_Couter2/3
  Equal30/1 -> Logical Operator22/4
  [VDDM_EPBUnlockTOCFSRls_flg] -> Switch1/2
  [VDDM_EPBUnlockTOCFS_flg] -> Logical Operator27/2
  Equal24/1 -> Logical Operator22/1
  [VINP_ShifterHandleCmd_enum] -> Equal25/1
  Constant38/1 -> Test Detection Criteria2/4
  Unit Delay1/1 -> Equal31/1
  Constant41/1 -> Equal24/2
  [DTC_clear_request] -> DTC_Info1/4
  SR_Latch5/1 -> Logical Operator24/2
  Data Type Conversion1/1 -> [VDDM_EPBUnlockTODTC_cnt]  "VDDM_EPBUnlockTODTC_cnt"
  Constant31/1 -> Logical Operator24/1
  Logical Operator13/1 -> DTC_Couter2/1
  Constant44/1 -> Logical Operator13/2
  DTC_Couter2/1 -> SR_Latch3/1
  Logical Operator17/1 -> DTC_Couter2/2
  Logical Operator18/1 -> [VDDM_EPBUnlockTOCFS_flg]  "VDDM_EPBUnlockTOCFS_flg"
  [VDDM_EPBUnlockTOCFS_flg] -> DTC_Info1/3
  Relay2/1 -> SR_Latch5/1
  DTC_Couter2/2 -> Data Type Conversion1/1
  [VDDM_EPBUnlockTOCFSRls_flg] -> Logical Operator10/3
  [VDDM_EPBUnlockTOPass_flg] -> Logical Operator10/2
  Constant36/1 -> Test Detection Criteria2/3
  [DTC_clear_request] -> Logical Operator20/3
  [VDDM_EPBUnlockTOCFSRls_flg] -> Logical Operator51/1
  Switch1/1 -> Test Detection Criteria2/1
  SR_Latch4/1 -> [VDDM_EPBUnlockTOPass_flg]  "VDDM_EPBUnlockTOPass_flg"
  Logical Operator24/1 -> [VDDM_EPBUnlockTODFS_flg]  "VDDM_EPBUnlockTODFS_flg"
  Logical Operator10/1 -> Logical Operator17/1
  DTC_Info1/1 -> VDDM_EPBUnlockTODTC_raw32/1  "VDDM_EPBUnlockTODTC_raw32"
  [VDDM_EPBUnlockTODet_flg] -> DTC_Info1/1
  [VDDM_EPBUnlockTODTC_cnt] -> Relay2/1
  [VDDM_EPBUnlockTODFSRls_flg] -> Logical Operator27/1
  Logical Operator7/1 -> Logical Operator6/1
  [VDDM_EPBLockTOPass_flg] -> Logical Operator6/2
  Constant17/1 -> Equal12/2
  Equal12/1 -> Logical Operator7/2
  [VINP_ShifterHandleCmd_enum] -> Equal14/1
  Logical Operator6/1 -> [VDDM_EPBLockTODFSRls_flg]  "VDDM_EPBLockTODFSRls_flg"
  Constant14/1 -> Equal11/2
  Equal11/1 -> Logical Operator7/1
  [VINP_ShifterHandleCmd_enum] -> Equal13/1
  [VINP_ShifterHandleCmd_enum] -> Equal11/1
  Equal14/1 -> Logical Operator7/4
  Constant19/1 -> Equal14/2
  [VINP_ShifterHandleCmd_enum] -> Equal12/1
  Equal13/1 -> Logical Operator7/3
  Constant18/1 -> Equal13/2
  [VINP_ShifterHandleCmd_enum] -> Equal8/1
  Logical Operator37/1 -> [VDDM_EPBLockTOCFSRls_flg]  "VDDM_EPBLockTOCFSRls_flg"
  Equal34/1 -> Logical Operator40/2
  [VINP_ShifterHandleCmd_enum] -> Equal34/1
  Equal6/1 -> Logical Operator40/3
  [VINP_ShifterHandleCmd_enum] -> Equal33/1
  Constant5/1 -> Equal8/2
  Logical Operator40/1 -> Logical Operator37/1
  Equal9/1 -> Logical Operator1/1
  Constant4/1 -> Equal6/2
  [VPMM_SysPwrSta_enum] -> Unit Delay4/1
  Equal8/1 -> Logical Operator40/4
  Constant13/1 -> Equal10/2
  Unit Delay4/1 -> Equal9/1
  [DTC_clear_request] -> Logical Operator37/3
  [VPMM_SysPwrSta_enum] -> Equal10/1
  Constant12/1 -> Equal9/2
  Constant46/1 -> Equal34/2
  [VINP_ShifterHandleCmd_enum] -> Equal6/1
  Equal33/1 -> Logical Operator40/1
  Logical Operator1/1 -> Logical Operator37/2
  Constant45/1 -> Equal33/2
  Equal10/1 -> Logical Operator1/2
  [VPMM_SysPwrSta_enum] -> Equal/1
  Constant/1 -> Equal/2
  Equal/1 -> Logical Operator/1
  Equal1/1 -> Logical Operator/2
  [NO_CAN1_BUS_OFF] -> Logical Operator3/1
  Logical Operator/1 -> Logical Operator3/5
  Constant8/1 -> Equal1/2
  [VDDM_EPBUnlockTOCFS_flg] -> Unit Delay/1
  [VPMM_SysPwrSta_enum] -> Equal1/1
  SR_Latch2/1 -> Logical Operator55/2
  Constant15/1 -> DTC_Couter1/3
  Logical Operator16/1 -> DTC_Couter1/2
  [VDDM_EPBLockTODet_flg] -> Logical Operator15/1
  [DTC_clear_request] -> DTC_Info/4
  Constant7/1 -> Logical Operator16/2
  [VDDM_EPBLockTOCFSRls_flg] -> Logical Operator11/3
  Constant1/1 -> Logical Operator2/2
  [VDDM_EPBLockTOPass_flg] -> Logical Operator11/2
  SR_Latch1/1 -> Logical Operator2/1
  Logical Operator11/1 -> Logical Operator16/1
  [VDDM_EPBLockTOCFSRls_flg] -> Switch6/2
  Logical Operator55/1 -> [VDDM_EPBLockTODFS_flg]  "VDDM_EPBLockTODFS_flg"
  Constant6/1 -> Logical Operator15/2
  Constant16/1 -> Logical Operator55/1
  Test Detection Criteria1/1 -> [VDDM_EPBLockTODet_flg]  "VDDM_EPBLockTODet_flg"
  DTC_Info/1 -> VDDM_EPBLockTODTC_raw32/1  "VDDM_EPBLockTODTC_raw32"
  Logical Operator77/1 -> SR_Latch2/2
  Relay1/1 -> SR_Latch2/1
  [task_time_s] -> Test Detection Criteria1/2
  [VDDM_EPBLockTODet_flg] -> DTC_Info/1
  [VDDM_EPBLockTOCFS_flg] -> DTC_Info/3
  DTC_Couter1/2 -> Data Type Conversion2/1
  Data Type Conversion2/1 -> [VDDM_EPBLockTODTC_cnt]  "VDDM_EPBLockTODTC_cnt"
  Constant20/1 -> Test Detection Criteria1/3
  Logical Operator2/1 -> [VDDM_EPBLockTOCFS_flg]  "VDDM_EPBLockTOCFS_flg"
  Constant2/1 -> Switch6/1
  [VDDM_EPBLockTOCFSRls_flg] -> Logical Operator49/1
  Constant22/1 -> Test Detection Criteria1/4
  Logical Operator3/1 -> Switch6/3, [VDDM_EPBLockTORst_flg]
  [VDDM_EPBLockTOPass_flg] -> DTC_Info/2
  Logical Operator15/1 -> DTC_Couter1/1
  DTC_Couter1/1 -> SR_Latch1/1
  [VDDM_EPBLockTODFSRls_flg] -> Logical Operator77/1
  Switch6/1 -> Test Detection Criteria1/1
  [VDDM_EPBLockTOCFS_flg] -> Logical Operator77/2
  [VDDM_EPBLockTODTC_cnt] -> Relay1/1
  [VDDM_EPBLockTODFS_flg] -> VDDM_EPBLockTODFS_flg/1
  [VDDM_EPBLockTOCFS_flg] -> VDDM_EPBLockTOCFS_flg/1
  [VDDM_EPBUnlockTODFS_flg] -> VDDM_EPBUnlockTODFS_flg/1
  [VDDM_EPBUnlockTOCFS_flg] -> VDDM_EPBUnlockTOCFS_flg/1
